simulink model "ControlLoopDiagrams"  (R2026a)
settings: Solver=VariableStepAuto
model workspace (MAT data in the model file):
  K = 1
  Kd = 1
  Kff = 1
  Ki = 1
  Kp = 1
  Kw = 1
  r = 1
libraries: simulink x1
settings Model: Creator=crefvem  LastModifiedBy=Charlie

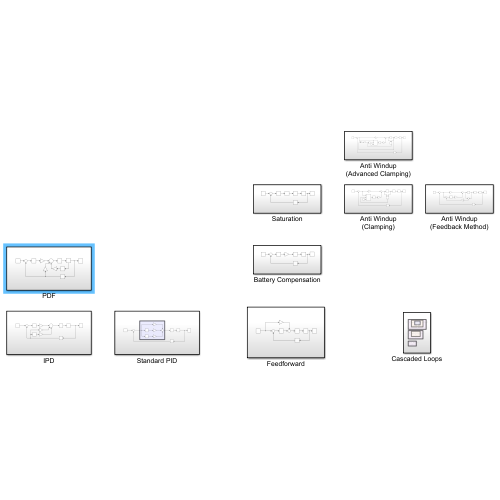
[thumbnail: Simulink's stored preview of the top-level diagram]
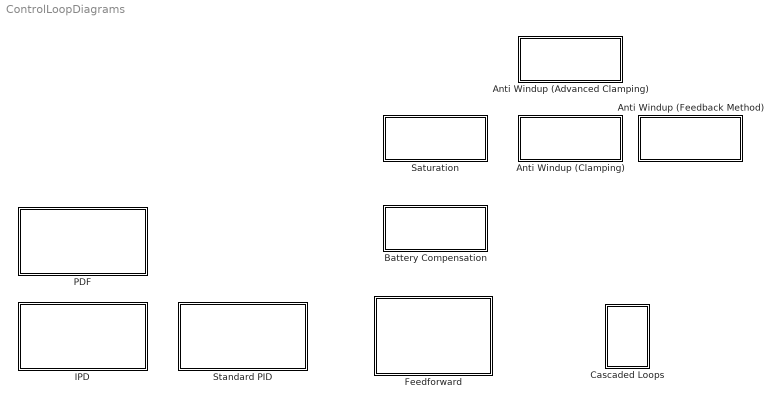
== system ControlLoopDiagrams ==
  Anti Windup (Advanced Clamping) : Subsystem
  Anti Windup (Clamping) : Subsystem
  Anti Windup (Feedback Method) : Subsystem
  Battery Compensation : Subsystem
  Cascaded Loops : Subsystem
  Feedforward : Subsystem
  IPD : Subsystem
  PDF : Subsystem
  Saturation : Subsystem
  Standard PID : Subsystem

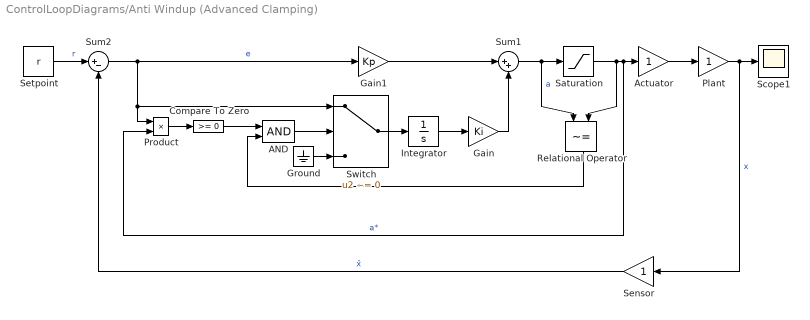
== system ControlLoopDiagrams/Anti Windup (Advanced Clamping) ==
  " Actuator " : Gain
      mask Display: disp('G_1', texmode="on")
  " Plant " : Gain
      mask Display: disp('G_2', texmode="on")
  " Sensor " : Gain
      mask Display: disp('H', texmode="on")
  " Setpoint " : Constant  Value=r
  AND : Logic  IconShape=distinctive  AllPortsSameDT=off  OutDataTypeStr=boolean
  Compare To Zero : simulink/Logic and Bit Operations/Compare To Zero  relop=>=  OutDataTypeStr=boolean
  Gain : Gain  Gain=Ki
  Gain1 : Gain  Gain=Kp
  Ground : Ground
  Integrator : Integrator
      mask Display: disp('\int dt', texmode="on")
  Product : Product
  Relational Operator : RelationalOperator  Operator=~=  OutDataTypeStr=boolean  RndMeth=Simplest  InputSameDT=off
  Saturation : Saturate
  Scope1 : Scope
      settings: DataLoggingVariableName=ScopeData5
  Sum1 : Sum  Inputs=|++
  Sum2 : Sum  Inputs=|+-
  Switch : Switch  Criteria=u2 ~= 0  SaturateOnIntegerOverflow=off  InputSameDT=off
  wires:
  " Plant "/1 -> " Sensor "/1, Scope1/1  "x"
  " Actuator "/1 -> " Plant "/1
  " Sensor "/1 -> Sum2/2  "x̂"
  " Setpoint "/1 -> Sum2/1  "r"
  Saturation/1 -> Product/2, " Actuator "/1, Relational Operator/2  "a*"
  Sum1/1 -> Saturation/1, Relational Operator/1  "a"
  Gain/1 -> Sum1/2
  Sum2/1 -> Gain1/1, Switch/1, Product/1  "e"
  Integrator/1 -> Gain/1
  Gain1/1 -> Sum1/1
  Relational Operator/1 -> AND/2
  Switch/1 -> Integrator/1
  Ground/1 -> Switch/3
  Product/1 -> Compare To Zero/1
  Compare To Zero/1 -> AND/1
  AND/1 -> Switch/2

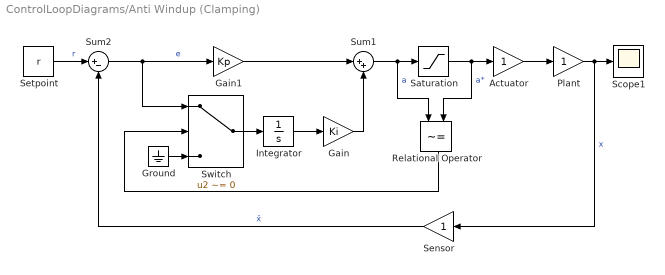
== system ControlLoopDiagrams/Anti Windup (Clamping) ==
  " Actuator " : Gain
      mask Display: disp('G_1', texmode="on")
  " Plant " : Gain
      mask Display: disp('G_2', texmode="on")
  " Sensor " : Gain
      mask Display: disp('H', texmode="on")
  " Setpoint " : Constant  Value=r
  Gain : Gain  Gain=Ki
  Gain1 : Gain  Gain=Kp
  Ground : Ground
  Integrator : Integrator
      mask Display: disp('\int dt', texmode="on")
  Relational Operator : RelationalOperator  Operator=~=  OutDataTypeStr=boolean  RndMeth=Simplest  InputSameDT=off
  Saturation : Saturate
  Scope1 : Scope
      settings: DataLoggingVariableName=ScopeData5
  Sum1 : Sum  Inputs=|++
  Sum2 : Sum  Inputs=|+-
  Switch : Switch  Criteria=u2 ~= 0  SaturateOnIntegerOverflow=off  InputSameDT=off
  wires:
  " Plant "/1 -> " Sensor "/1, Scope1/1  "x"
  " Actuator "/1 -> " Plant "/1
  " Sensor "/1 -> Sum2/2  "x̂"
  " Setpoint "/1 -> Sum2/1  "r"
  Saturation/1 -> " Actuator "/1, Relational Operator/2  "a*"
  Sum1/1 -> Relational Operator/1, Saturation/1  "a"
  Gain/1 -> Sum1/2
  Sum2/1 -> Gain1/1, Switch/1  "e"
  Integrator/1 -> Gain/1
  Gain1/1 -> Sum1/1
  Switch/1 -> Integrator/1
  Ground/1 -> Switch/3
  Relational Operator/1 -> Switch/2

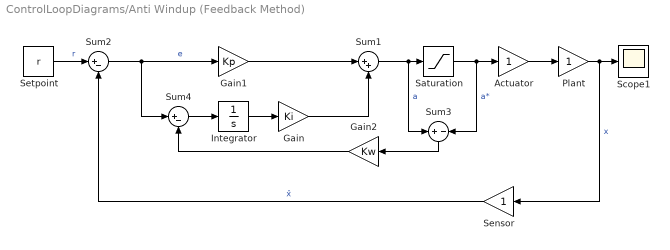
== system ControlLoopDiagrams/Anti Windup (Feedback Method) ==
  " Actuator " : Gain
      mask Display: disp('G_1', texmode="on")
  " Plant " : Gain
      mask Display: disp('G_2', texmode="on")
  " Sensor " : Gain
      mask Display: disp('H', texmode="on")
  " Setpoint " : Constant  Value=r
  Gain : Gain  Gain=Ki
  Gain1 : Gain  Gain=Kp
  Gain2 : Gain  Gain=Kw
  Integrator : Integrator
      mask Display: disp('\int dt', texmode="on")
  Saturation : Saturate
  Scope1 : Scope
      settings: DataLoggingVariableName=ScopeData5
  Sum1 : Sum  Inputs=|++
  Sum2 : Sum  Inputs=|+-
  Sum3 : Sum  Inputs=+|-
  Sum4 : Sum  Inputs=|+-
  wires:
  Sum4/1 -> Integrator/1
  Gain1/1 -> Sum1/1
  Integrator/1 -> Gain/1
  Sum2/1 -> Sum4/1, Gain1/1  "e"
  Gain/1 -> Sum1/2
  Sum1/1 -> Sum3/1, Saturation/1  "a"
  Saturation/1 -> Sum3/2, " Actuator "/1  "a*"
  " Setpoint "/1 -> Sum2/1  "r"
  " Sensor "/1 -> Sum2/2  "x̂"
  " Actuator "/1 -> " Plant "/1
  " Plant "/1 -> Scope1/1, " Sensor "/1  "x"
  Sum3/1 -> Gain2/1
  Gain2/1 -> Sum4/2

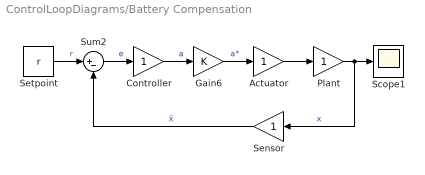
== system ControlLoopDiagrams/Battery Compensation ==
  " Actuator " : Gain
      mask Display: disp('G_1', texmode="on")
  " Controller " : Gain
      mask Display: disp('C', texmode="on")
  " Plant " : Gain
      mask Display: disp('G_2', texmode="on")
  " Sensor " : Gain
      mask Display: disp('H', texmode="on")
  " Setpoint " : Constant  Value=r
  Gain6 : Gain  Gain=K
  Scope1 : Scope
      settings: DataLoggingVariableName=ScopeData5
  Sum2 : Sum  Inputs=|+-
  wires:
  " Controller "/1 -> Gain6/1  "a"
  Gain6/1 -> " Actuator "/1  "a*"
  " Setpoint "/1 -> Sum2/1  "r"
  " Sensor "/1 -> Sum2/2  "x̂"
  " Actuator "/1 -> " Plant "/1
  Sum2/1 -> " Controller "/1  "e"
  " Plant "/1 -> Scope1/1, " Sensor "/1  "x"

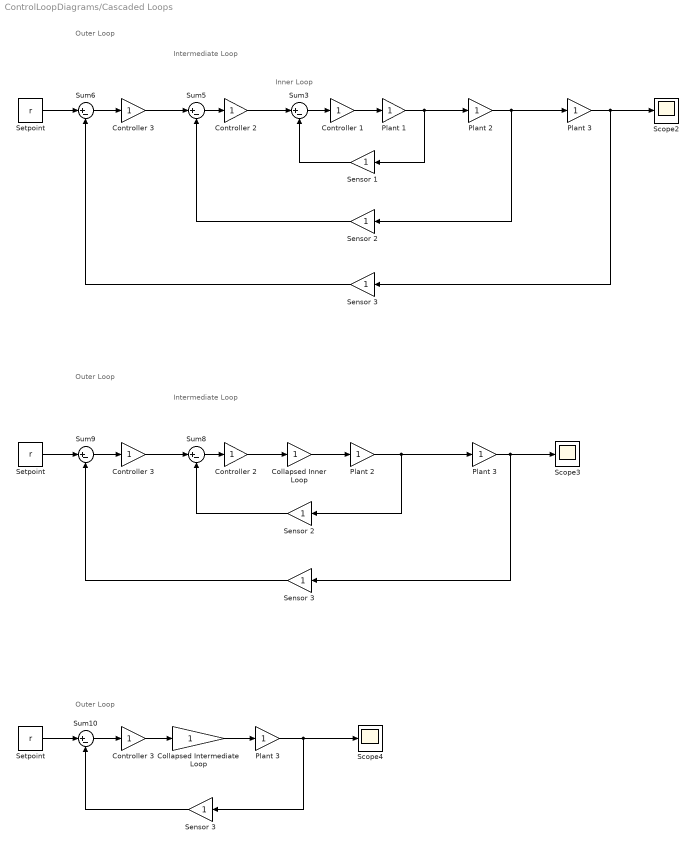
== system ControlLoopDiagrams/Cascaded Loops ==
  note: Outer Loop
  note: Intermediate Loop
  note: Inner Loop
  note: Outer Loop
  note: Intermediate Loop
  note: Outer Loop
  "    Setpoint    " : Constant  Value=r
  "   Setpoint   " : Constant  Value=r
  "  Controller 3  " : Gain
      mask Display: disp('C_3', texmode="on")
  "  Plant 3  " : Gain
      mask Display: disp('G_3', texmode="on")
  "  Sensor 3  " : Gain
      mask Display: disp('H_3', texmode="on")
  "  Setpoint  " : Constant  Value=r
  " Controller 2 " : Gain
      mask Display: disp('C_2', texmode="on")
  " Controller 3 " : Gain
      mask Display: disp('C_3', texmode="on")
  " Plant 2 " : Gain
      mask Display: disp('G_2', texmode="on")
  " Plant 3 " : Gain
      mask Display: disp('G_3', texmode="on")
  " Sensor 2 " : Gain
      mask Display: disp('H_2', texmode="on")
  " Sensor 3 " : Gain
      mask Display: disp('H_3', texmode="on")
  Collapsed Inner Loop : Gain
      mask Display: disp('G_{inner}', texmode="on")
  Collapsed Intermediate Loop : Gain
      mask Display: disp('G_{intermediate}', texmode="on")
  Controller 1 : Gain
      mask Display: disp('C_1', texmode="on")
  Controller 2 : Gain
      mask Display: disp('C_2', texmode="on")
  Controller 3 : Gain
      mask Display: disp('C_3', texmode="on")
  Plant 1 : Gain
      mask Display: disp('G_1', texmode="on")
  Plant 2 : Gain
      mask Display: disp('G_2', texmode="on")
  Plant 3 : Gain
      mask Display: disp('G_3', texmode="on")
  Scope2 : Scope
      settings: DataLoggingVariableName=ScopeData2
  Scope3 : Scope
      settings: DataLoggingVariableName=ScopeData3
  Scope4 : Scope
      settings: DataLoggingVariableName=ScopeData4
  Sensor 1 : Gain
      mask Display: disp('H_1', texmode="on")
  Sensor 2 : Gain
      mask Display: disp('H_2', texmode="on")
  Sensor 3 : Gain
      mask Display: disp('H_3', texmode="on")
  Sum{3,5..6,8..10} (6 alike) : Sum  Inputs=|+-
  wires:
  Collapsed Inner Loop/1 -> " Plant 2 "/1
  Sum6/1 -> Controller 3/1
  " Sensor 2 "/1 -> Sum8/2
  "  Plant 3  "/1 -> "  Sensor 3  "/1, Scope4/1
  " Sensor 3 "/1 -> Sum9/2
  Collapsed Intermediate Loop/1 -> "  Plant 3  "/1
  "   Setpoint   "/1 -> Sum9/1
  " Plant 2 "/1 -> " Sensor 2 "/1, " Plant 3 "/1
  Sum10/1 -> "  Controller 3  "/1
  Sum8/1 -> " Controller 2 "/1
  "  Sensor 3  "/1 -> Sum10/2
  Plant 3/1 -> Scope2/1, Sensor 3/1
  Controller 1/1 -> Plant 1/1
  Sum5/1 -> Controller 2/1
  Plant 1/1 -> Plant 2/1, Sensor 1/1
  Controller 2/1 -> Sum3/1
  " Controller 2 "/1 -> Collapsed Inner Loop/1
  Sensor 3/1 -> Sum6/2
  "    Setpoint    "/1 -> Sum10/1
  Sensor 1/1 -> Sum3/2
  " Controller 3 "/1 -> Sum8/1
  Controller 3/1 -> Sum5/1
  " Plant 3 "/1 -> " Sensor 3 "/1, Scope3/1
  Plant 2/1 -> Plant 3/1, Sensor 2/1
  "  Setpoint  "/1 -> Sum6/1
  Sensor 2/1 -> Sum5/2
  "  Controller 3  "/1 -> Collapsed Intermediate Loop/1
  Sum9/1 -> " Controller 3 "/1
  Sum3/1 -> Controller 1/1

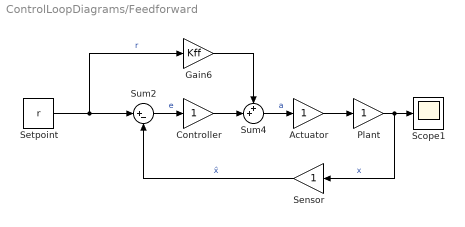
== system ControlLoopDiagrams/Feedforward ==
  " Actuator " : Gain
      mask Display: disp('G_1', texmode="on")
  " Controller " : Gain
      mask Display: disp('C', texmode="on")
  " Plant " : Gain
      mask Display: disp('G_2', texmode="on")
  " Sensor " : Gain
      mask Display: disp('H', texmode="on")
  " Setpoint " : Constant  Value=r
  Gain6 : Gain  Gain=Kff
  Scope1 : Scope
  Sum2 : Sum  Inputs=|+-
  Sum4 : Sum  Inputs=++|
  wires:
  " Plant "/1 -> Scope1/1, " Sensor "/1  "x"
  Sum2/1 -> " Controller "/1  "e"
  Gain6/1 -> Sum4/1
  " Sensor "/1 -> Sum2/2  "x̂"
  " Actuator "/1 -> " Plant "/1
  Sum4/1 -> " Actuator "/1  "a"
  " Setpoint "/1 -> Gain6/1, Sum2/1  "r"
  " Controller "/1 -> Sum4/2

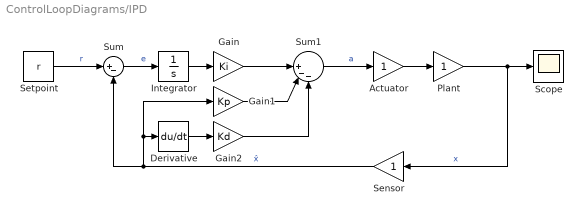
== system ControlLoopDiagrams/IPD ==
  Actuator : Gain
      mask Display: disp('G_1', texmode="on")
  Derivative : Derivative
      mask Display: disp('{d}/{dt}', texmode="on")
  Gain : Gain  Gain=Ki
  Gain1 : Gain  Gain=Kp
  Gain2 : Gain  Gain=Kd
  Integrator : Integrator
      mask Display: disp('\int dt', texmode="on")
  Plant : Gain
      mask Display: disp('G_2', texmode="on")
  Scope : Scope
  Sensor : Gain
      mask Display: disp('H', texmode="on")
  Setpoint : Constant  Value=r
  Sum : Sum  Inputs=|+-
  Sum1 : Sum  Inputs=||+--
  wires:
  Actuator/1 -> Plant/1
  Plant/1 -> Sensor/1, Scope/1  "x"
  Sum1/1 -> Actuator/1  "a"
  Integrator/1 -> Gain/1
  Sensor/1 -> Sum/2, Gain1/1, Derivative/1  "x̂"
  Gain2/1 -> Sum1/3
  Gain/1 -> Sum1/1
  Setpoint/1 -> Sum/1  "r"
  Gain1/1 -> Sum1/2
  Sum/1 -> Integrator/1  "e"
  Derivative/1 -> Gain2/1

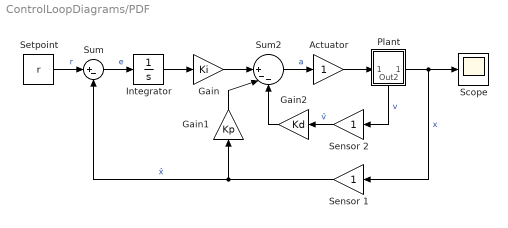
== system ControlLoopDiagrams/PDF ==
  Actuator : Gain
      mask Display: disp('G_1', texmode="on")
  Gain : Gain  Gain=Ki
  Gain1 : Gain  Gain=Kp
  Gain2 : Gain  Gain=Kd
  Integrator : Integrator
      mask Display: disp('\int dt', texmode="on")
  Plant : Subsystem
      settings: PortSchema="{\"entries\":[{\"content\":{\"sides\":[{\"content\":{\"connectorIds\":[\"In1\"]},\"type\":\"ConnectorPlacement.EquallySpacedRectSide\",\"uuid\":\"01b4b555-e57c-46dc-bbdd-6c047e3bac1e\"},{\"content\":{\"connectorIds\":[\"Out1\"],\"side\":\"RIGHT\"},\"type\":\"ConnectorPlacement.EquallySpacedRectSide\",\"uuid\":\"5cfdd333-c627-47b1-b231-0f4db4765b56\"},{\"content\":{\"side\":\"TOP\"},\"type\":\"ConnectorPlacement.EquallySpacedRectSide\",\"uuid\":\"bc9a65da-f4b1-4adc-939b-4522115df914\"},{\"content\":{\"connectorIds\":[\"Out2\"],\"side\":\"BOTTOM\"},\"type\":\"ConnectorPlacement.EquallySpacedRectSide\",\"uuid\":\"4beef4a5-00cd-423f-8bb5-dc02d5ccbdaf\"}]},\"type\":\"ConnectorPlacement.EquallySpacedConnector\",\"uuid\":\"cdc21ac0-2f2c-4db8-baa2-e971ea05d0d4\"}],\"packageUris\":[\"http://schema.mathworks.com/mf0/Connector/R2020b\"],\"version\":\"1.0\"}"
      mask Display: disp('G_2', texmode="on")
  Scope : Scope
  Sensor 1 : Gain
      mask Display: disp('H_1', texmode="on")
  Sensor 2 : Gain
      mask Display: disp('H_2', texmode="on")
  Setpoint : Constant  Value=r
  Sum : Sum  Inputs=|+-
  Sum2 : Sum  Inputs=||+--
  wires:
  Sensor 2/1 -> Gain2/1  "v̂"
  Sum/1 -> Integrator/1  "e"
  Gain1/1 -> Sum2/2
  Setpoint/1 -> Sum/1  "r"
  Gain2/1 -> Sum2/3
  Sensor 1/1 -> Sum/2, Gain1/1  "x̂"
  Integrator/1 -> Gain/1
  Sum2/1 -> Actuator/1  "a"
  Plant/1(Out1) -> Scope/1, Sensor 1/1  "x"
  Actuator/1 -> Plant/1(In1)
  Gain/1 -> Sum2/1
  Plant/2(Out2) -> Sensor 2/1  "v"

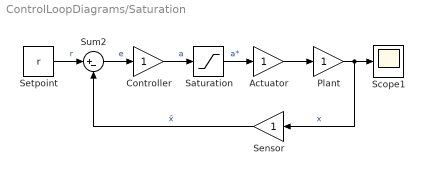
== system ControlLoopDiagrams/Saturation ==
  " Actuator " : Gain
      mask Display: disp('G_1', texmode="on")
  " Controller " : Gain
      mask Display: disp('C', texmode="on")
  " Plant " : Gain
      mask Display: disp('G_2', texmode="on")
  " Sensor " : Gain
      mask Display: disp('H', texmode="on")
  " Setpoint " : Constant  Value=r
  Saturation : Saturate
  Scope1 : Scope
      settings: DataLoggingVariableName=ScopeData5
  Sum2 : Sum  Inputs=|+-
  wires:
  " Controller "/1 -> Saturation/1  "a"
  Saturation/1 -> " Actuator "/1  "a*"
  " Setpoint "/1 -> Sum2/1  "r"
  " Sensor "/1 -> Sum2/2  "x̂"
  " Actuator "/1 -> " Plant "/1
  Sum2/1 -> " Controller "/1  "e"
  " Plant "/1 -> Scope1/1, " Sensor "/1  "x"

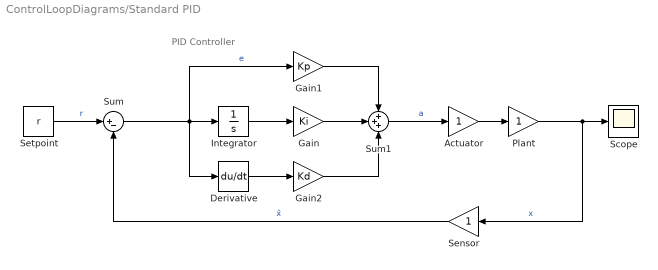
== system ControlLoopDiagrams/Standard PID ==
  note: PID Controller
  Actuator : Gain
      mask Display: disp('G_1', texmode="on")
  Derivative : Derivative
      mask Display: disp('{d}/{dt}', texmode="on")
  Gain : Gain  Gain=Ki
  Gain1 : Gain  Gain=Kp
  Gain2 : Gain  Gain=Kd
  Integrator : Integrator
      mask Display: disp('\int dt', texmode="on")
  Plant : Gain
      mask Display: disp('G_2', texmode="on")
  Scope : Scope
  Sensor : Gain
      mask Display: disp('H', texmode="on")
  Setpoint : Constant  Value=r
  Sum : Sum  Inputs=|+-
  Sum1 : Sum  Inputs=+++
  wires:
  Derivative/1 -> Gain2/1
  Sum/1 -> Gain1/1, Derivative/1, Integrator/1  "e"
  Gain1/1 -> Sum1/1
  Setpoint/1 -> Sum/1  "r"
  Gain/1 -> Sum1/2
  Gain2/1 -> Sum1/3
  Sensor/1 -> Sum/2  "x̂"
  Integrator/1 -> Gain/1
  Sum1/1 -> Actuator/1  "a"
  Plant/1 -> Scope/1, Sensor/1  "x"
  Actuator/1 -> Plant/1

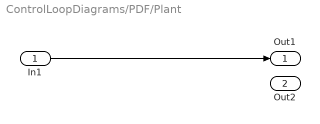
== system ControlLoopDiagrams/PDF/Plant ==
  In1 : Inport
  Out1 : Outport
  Out2 : Outport  Port=2
  wires:
  In1/1 -> Out1/1
